simulink model "DIL_26_5_1_2023b"  (R2023b)
settings: Solver=FixedStepAuto  StartTime=0.0  StopTime=inf  FixedStep=0.0005  RelTol=1e-3
PostLoadFcn:
  | modelDir = fileparts(get_param(bdroot,'FileName')); if ~contains([path pathsep],[modelDir pathsep]), addpath(modelDir); end
libraries: Solver_SF x1, slpidlib x1, sl3dlib x1
settings Model: LastModifiedBy=30235
settings SolverCC: AlgebraicLoopSolver=TrustRegion
settings OptimizationCC: DefaultParameterBehavior=Inlined  OptimizeBlockIOStorage=off  EnhancedBackFolding=on  PassReuseOutputArgsThreshold=0  OptimizeDataStoreBuffers=off  BusAssignmentInplaceUpdate=off
settings DebuggingCC: ParameterTunabilityLossMsg=error  UnconnectedInputMsg=warning  UnconnectedOutputMsg=warning  UnconnectedLineMsg=warning  SFUnexpectedBacktrackingDiag=warning  SFNoUnconditionalDefaultTransitionDiag=warning  ArithmeticOperatorsInVariantConditions=warning
settings ModelReferenceCC: EnableRefExpFcnMdlSchedulingChecks=on
settings SFSimCC: MATLABDynamicMemAlloc=off  CustomCodeUndefinedFunction=UseInterfaceOnly
settings RTWCC: GenerateReport=on  BuildConfiguration=Debug  LaunchReport=on  DLArmComputeVersion=19.05
settings CodeAppCC: ForceParamTrailComments=on  OperatorAnnotations=on  MATLABSourceComments=on  EnableCustomComments=on
settings GRTTargetCC: CombineSignalStateStructs=on  SupportVariableSizeSignals=on  MultiInstanceErrorCode=Warning
settings ConfigComp: CovBoundaryAbsTol=1.0e-5

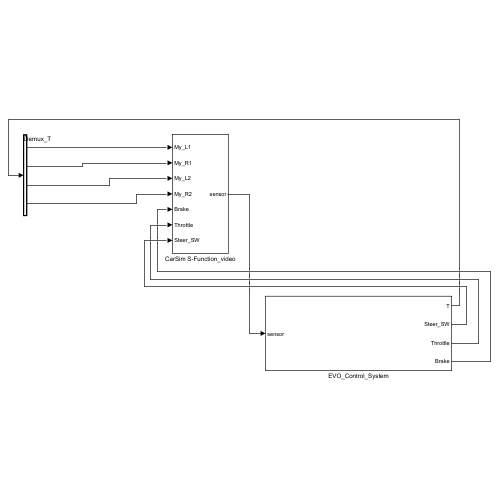
[thumbnail: Simulink's stored preview of the top-level diagram]
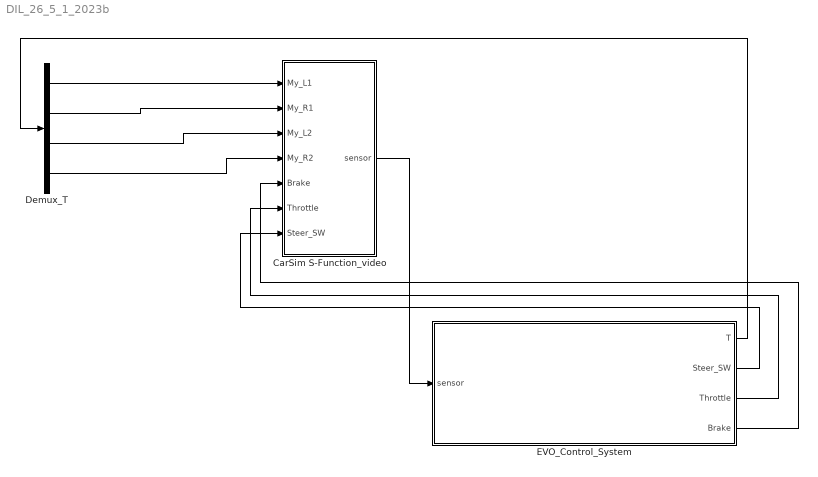
== system DIL_26_5_1_2023b ==
  CarSim S-Function_video : Subsystem
  Demux_T : Demux
  EVO_Control_System : Subsystem
  wires:
  EVO_Control_System/1(T) -> Demux_T/1
  Demux_T/1 -> CarSim S-Function_video/1(My_L1)
  Demux_T/2 -> CarSim S-Function_video/2(My_R1)
  Demux_T/3 -> CarSim S-Function_video/3(My_L2)
  Demux_T/4 -> CarSim S-Function_video/4(My_R2)
  EVO_Control_System/4(Brake) -> CarSim S-Function_video/5(Brake)
  EVO_Control_System/3(Throttle) -> CarSim S-Function_video/6(Throttle)
  EVO_Control_System/2(Steer_SW) -> CarSim S-Function_video/7(Steer_SW)
  CarSim S-Function_video/1(sensor) -> EVO_Control_System/1(sensor)

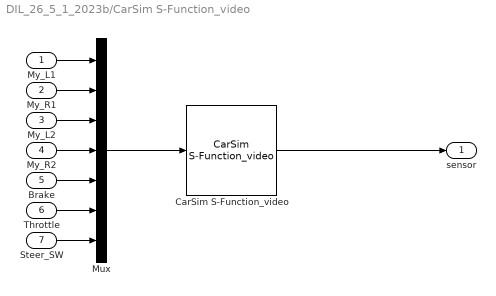
== system DIL_26_5_1_2023b/CarSim S-Function_video ==
  My_L1 : Inport
  My_R1 : Inport  Port=2
  My_L2 : Inport  Port=3
  My_R2 : Inport  Port=4
  Brake : Inport  Port=5
  Throttle : Inport  Port=6
  Steer_SW : Inport  Port=7
  CarSim S-Function_video : Solver_SF/CarSim S-Function_video  Priority=1  SIMFILE=simfile.sim
      settings: SourceProductName=CarSim S-Function
  Mux : Mux  Inputs=7
  sensor : Outport
  wires:
  CarSim S-Function_video/1 -> sensor/1
  My_L1/1 -> Mux/1
  My_R1/1 -> Mux/2
  My_L2/1 -> Mux/3
  My_R2/1 -> Mux/4
  Brake/1 -> Mux/5
  Throttle/1 -> Mux/6
  Steer_SW/1 -> Mux/7
  Mux/1 -> CarSim S-Function_video/1

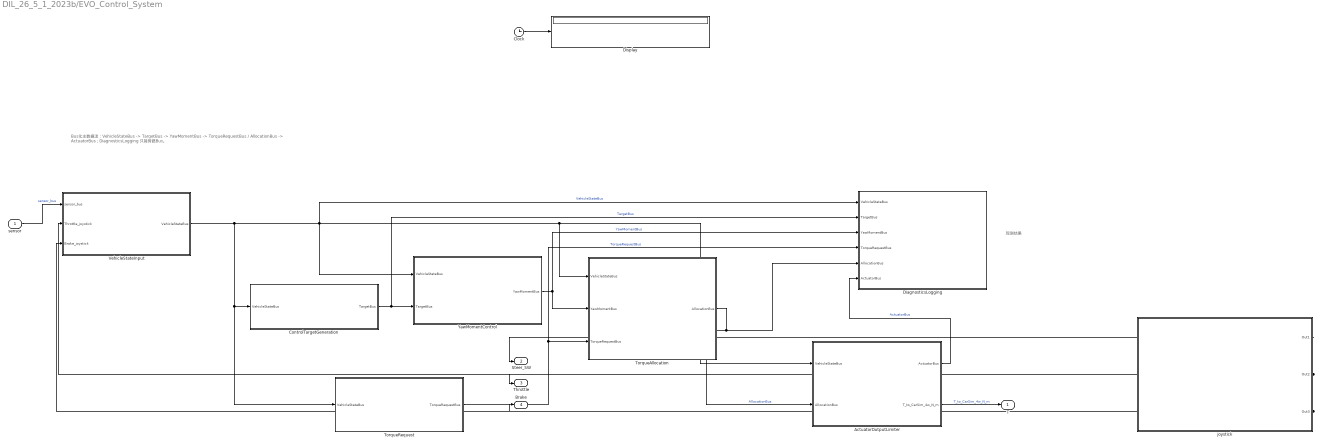
== system DIL_26_5_1_2023b/EVO_Control_System ==
  note: 观测结果
  note: Bus化主数据流：VehicleStateBus -> TargetBus -> YawMomentBus -> TorqueRequestBus / AllocationBus -> ActuatorBus；DiagnosticsLogging 只接旁路Bus。
  sensor : Inport
  ActuatorOutputLimiter : Subsystem  Description=执行器输出限制：统一执行电机转速限扭、最终饱和和传动输出。
  Clock : Clock
  ControlTargetGeneration : Subsystem  Description=控制目标生成：根据车辆状态和转角生成理想侧偏角与理想横摆角速度。
  DiagnosticsLogging : Subsystem  Description=诊断记录：集中显示基础扭矩、DYC 增量、QP 诊断和最终限扭差值。
  Display : Display
  TorqueAllocation : Subsystem  Description=转矩分配：保留简化载荷转移分配和 QP 分配，并通过 TorqueAllocationMode 选择。
  TorqueRequest : Subsystem  Description=基础扭矩请求：根据油门和制动状态生成控制分配层使用的基础扭矩。
  VehicleStateInput : Subsystem  Description=车辆状态输入整理：CarSim sensor 拆分、单位转换、轮胎力估算和基础状态 tag 输出。
  YawMomentControl : Subsystem  Description=横摆力矩控制：保留 PID 与 MPC 两条路径，并通过 YawMomentControlMode 选择。
  joystick : Subsystem
  T : Outport
  Steer_SW : Outport  Port=2
  Throttle : Outport  Port=3
  Brake : Outport  Port=4
  wires:
  sensor/1 -> VehicleStateInput/1(sensor_bus)  "sensor_bus"
  TorqueAllocation/1(AllocationBus) -> ActuatorOutputLimiter/2(AllocationBus), DiagnosticsLogging/5(AllocationBus)  "AllocationBus"
  VehicleStateInput/1(VehicleStateBus) -> ActuatorOutputLimiter/1(VehicleStateBus), TorqueAllocation/1(VehicleStateBus), DiagnosticsLogging/1(VehicleStateBus), YawMomentControl/1(VehicleStateBus), ControlTargetGeneration/1(VehicleStateBus), TorqueRequest/1(VehicleStateBus)  "VehicleStateBus"
  ControlTargetGeneration/1(TargetBus) -> YawMomentControl/2(TargetBus), DiagnosticsLogging/2(TargetBus)  "TargetBus"
  ActuatorOutputLimiter/2(T_to_CarSim_4w_N_m) -> T/1  "T_to_CarSim_4w_N_m"
  ActuatorOutputLimiter/1(ActuatorBus) -> DiagnosticsLogging/6(ActuatorBus)  "ActuatorBus"
  YawMomentControl/1(YawMomentBus) -> DiagnosticsLogging/3(YawMomentBus), TorqueAllocation/2(YawMomentBus)  "YawMomentBus"
  TorqueRequest/1(TorqueRequestBus) -> DiagnosticsLogging/4(TorqueRequestBus), TorqueAllocation/3(TorqueRequestBus)  "TorqueRequestBus"
  Clock/1 -> Display/1
  joystick/1(Out1) -> Steer_SW/1
  joystick/2(Out2) -> Throttle/1, VehicleStateInput/2(Throttle_joystick)
  joystick/3(Out3) -> Brake/1, VehicleStateInput/3(Brake_joystick)

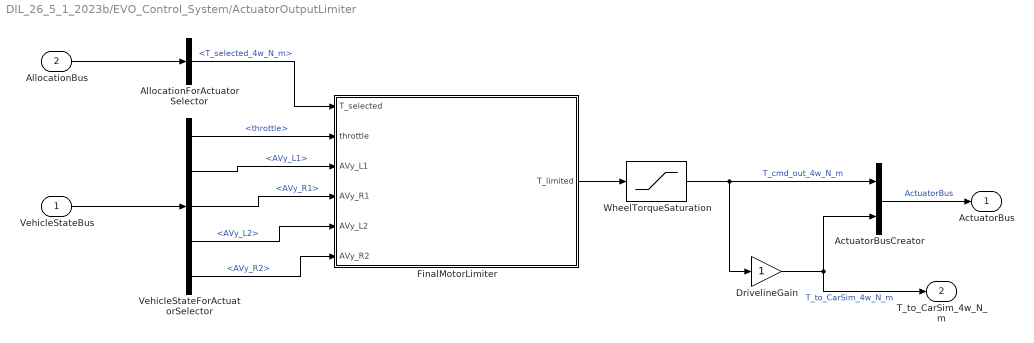
== system DIL_26_5_1_2023b/EVO_Control_System/ActuatorOutputLimiter ==
  VehicleStateBus : Inport
  AllocationBus : Inport  Port=2
  ActuatorBusCreator : BusCreator  Inputs=2
      settings: DisplayOption=signals
  AllocationForActuatorSelector : BusSelector  OutputSignals=T_selected_4w_N_m
  DrivelineGain : Gain
  FinalMotorLimiter : MATLAB Function  TreatAsAtomicUnit=on
  VehicleStateForActuatorSelector : BusSelector  OutputSignals=throttle,AVy_L1,AVy_R1,AVy_L2,AVy_R2
  WheelTorqueSaturation : Saturate  UpperLimit=400  LowerLimit=-400
  ActuatorBus : Outport
  T_to_CarSim_4w_N_m : Outport  Port=2
  wires:
  AllocationBus/1 -> AllocationForActuatorSelector/1
  VehicleStateBus/1 -> VehicleStateForActuatorSelector/1
  AllocationForActuatorSelector/1 -> FinalMotorLimiter/1(T_selected)  "<T_selected_4w_N_m>"
  VehicleStateForActuatorSelector/4 -> FinalMotorLimiter/5(AVy_L2)  "<AVy_L2>"
  VehicleStateForActuatorSelector/2 -> FinalMotorLimiter/3(AVy_L1)  "<AVy_L1>"
  VehicleStateForActuatorSelector/1 -> FinalMotorLimiter/2(throttle)  "<throttle>"
  VehicleStateForActuatorSelector/3 -> FinalMotorLimiter/4(AVy_R1)  "<AVy_R1>"
  VehicleStateForActuatorSelector/5 -> FinalMotorLimiter/6(AVy_R2)  "<AVy_R2>"
  FinalMotorLimiter/1(T_limited) -> WheelTorqueSaturation/1
  WheelTorqueSaturation/1 -> ActuatorBusCreator/1, DrivelineGain/1  "T_cmd_out_4w_N_m"
  DrivelineGain/1 -> ActuatorBusCreator/2, T_to_CarSim_4w_N_m/1  "T_to_CarSim_4w_N_m"
  ActuatorBusCreator/1 -> ActuatorBus/1  "ActuatorBus"

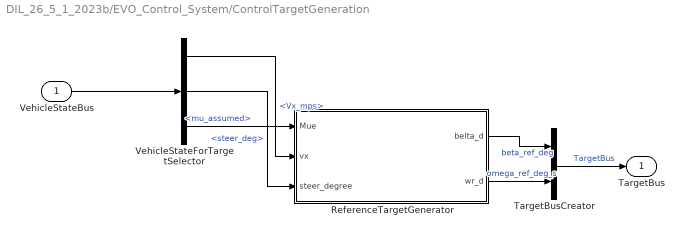
== system DIL_26_5_1_2023b/EVO_Control_System/ControlTargetGeneration ==
  VehicleStateBus : Inport
  ReferenceTargetGenerator : MATLAB Function  TreatAsAtomicUnit=on
  TargetBusCreator : BusCreator  Inputs=2
      settings: DisplayOption=signals
  VehicleStateForTargetSelector : BusSelector  OutputSignals=Vx_mps,steer_deg,mu_assumed
  TargetBus : Outport
  wires:
  VehicleStateForTargetSelector/3 -> ReferenceTargetGenerator/1(Mue)  "<mu_assumed>"
  VehicleStateForTargetSelector/2 -> ReferenceTargetGenerator/3(steer_degree)  "<steer_deg>"
  VehicleStateBus/1 -> VehicleStateForTargetSelector/1
  TargetBusCreator/1 -> TargetBus/1  "TargetBus"
  VehicleStateForTargetSelector/1 -> ReferenceTargetGenerator/2(vx)  "<Vx_mps>"
  ReferenceTargetGenerator/1(belta_d) -> TargetBusCreator/1  "beta_ref_deg"
  ReferenceTargetGenerator/2(wr_d) -> TargetBusCreator/2  "omega_ref_deg_s"

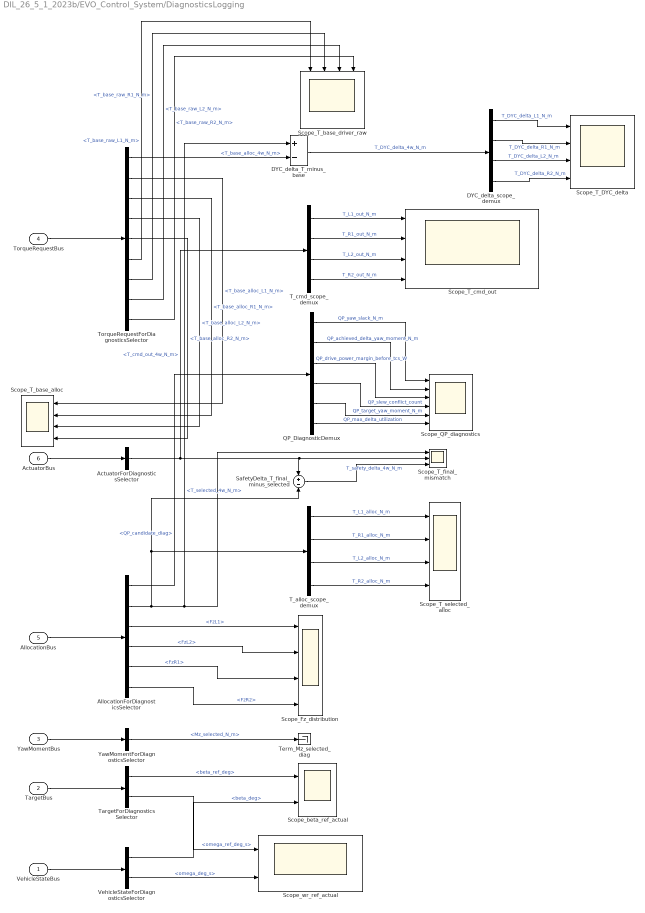
== system DIL_26_5_1_2023b/EVO_Control_System/DiagnosticsLogging ==
  VehicleStateBus : Inport
  TargetBus : Inport  Port=2
  YawMomentBus : Inport  Port=3
  TorqueRequestBus : Inport  Port=4
  AllocationBus : Inport  Port=5
  ActuatorBus : Inport  Port=6
  ActuatorForDiagnosticsSelector : BusSelector  OutputSignals=T_cmd_out_4w_N_m
  AllocationForDiagnosticsSelector : BusSelector  OutputSignals=QP_candidate_diag,T_selected_4w_N_m,FzL1,FzL2,FzR1,FzR2
  DYC_delta_T_minus_base : Sum  Inputs=+-
  DYC_delta_scope_demux : Demux
  QP_DiagnosticDemux : Demux  Outputs=6
  SafetyDelta_T_final_minus_selected : Sum  Inputs=+-
  Scope_Fz_distribution : Scope  NumInputPorts=4
  Scope_QP_diagnostics : Scope  NumInputPorts=6
  Scope_T_DYC_delta : Scope  NumInputPorts=4
  Scope_T_base_alloc : Scope  NumInputPorts=4
  Scope_T_base_driver_raw : Scope  NumInputPorts=4
  Scope_T_cmd_out : Scope  NumInputPorts=4
  Scope_T_final_mismatch : Scope  NumInputPorts=3
  Scope_T_selected_alloc : Scope  NumInputPorts=4
  Scope_beta_ref_actual : Scope  NumInputPorts=2
  Scope_wr_ref_actual : Scope  NumInputPorts=2
  T_alloc_scope_demux : Demux
  T_cmd_scope_demux : Demux
  TargetForDiagnosticsSelector : BusSelector  OutputSignals=beta_ref_deg,omega_ref_deg_s
  Term_Mz_selected_diag : Terminator
  TorqueRequestForDiagnosticsSelector : BusSelector  OutputSignals=T_base_alloc_4w_N_m,T_base_alloc_L1_N_m,T_base_alloc_R1_N_m,T_base_alloc_L2_N_m,T_base_alloc_R2_N_m,T_base_raw_L1_N_m,T_base_raw_R1_N_m,T_base_raw_L2_N_m,T_base_raw_R2_N_m
  VehicleStateForDiagnosticsSelector : BusSelector  OutputSignals=beta_deg,omega_deg_s
  YawMomentForDiagnosticsSelector : BusSelector  OutputSignals=Mz_selected_N_m
  wires:
  QP_DiagnosticDemux/3 -> Scope_QP_diagnostics/3  "QP_drive_power_margin_before_tcs_W"
  ActuatorBus/1 -> ActuatorForDiagnosticsSelector/1
  TorqueRequestBus/1 -> TorqueRequestForDiagnosticsSelector/1
  AllocationForDiagnosticsSelector/3 -> Scope_Fz_distribution/1  "<FzL1>"
  AllocationBus/1 -> AllocationForDiagnosticsSelector/1
  YawMomentBus/1 -> YawMomentForDiagnosticsSelector/1
  T_alloc_scope_demux/1 -> Scope_T_selected_alloc/1  "T_L1_alloc_N_m"
  T_cmd_scope_demux/3 -> Scope_T_cmd_out/3  "T_L2_out_N_m"
  TargetBus/1 -> TargetForDiagnosticsSelector/1
  DYC_delta_scope_demux/1 -> Scope_T_DYC_delta/1  "T_DYC_delta_L1_N_m"
  VehicleStateBus/1 -> VehicleStateForDiagnosticsSelector/1
  TorqueRequestForDiagnosticsSelector/2 -> Scope_T_base_alloc/1  "<T_base_alloc_L1_N_m>"
  DYC_delta_scope_demux/4 -> Scope_T_DYC_delta/4  "T_DYC_delta_R2_N_m"
  TorqueRequestForDiagnosticsSelector/9 -> Scope_T_base_driver_raw/4  "<T_base_raw_R2_N_m>"
  TorqueRequestForDiagnosticsSelector/1 -> DYC_delta_T_minus_base/2  "<T_base_alloc_4w_N_m>"
  TorqueRequestForDiagnosticsSelector/3 -> Scope_T_base_alloc/2  "<T_base_alloc_R1_N_m>"
  VehicleStateForDiagnosticsSelector/1 -> Scope_beta_ref_actual/2  "<beta_deg>"
  TorqueRequestForDiagnosticsSelector/4 -> Scope_T_base_alloc/3  "<T_base_alloc_L2_N_m>"
  VehicleStateForDiagnosticsSelector/2 -> Scope_wr_ref_actual/2  "<omega_deg_s>"
  TorqueRequestForDiagnosticsSelector/5 -> Scope_T_base_alloc/4  "<T_base_alloc_R2_N_m>"
  TorqueRequestForDiagnosticsSelector/6 -> Scope_T_base_driver_raw/1  "<T_base_raw_L1_N_m>"
  TorqueRequestForDiagnosticsSelector/7 -> Scope_T_base_driver_raw/2  "<T_base_raw_R1_N_m>"
  YawMomentForDiagnosticsSelector/1 -> Term_Mz_selected_diag/1  "<Mz_selected_N_m>"
  TorqueRequestForDiagnosticsSelector/8 -> Scope_T_base_driver_raw/3  "<T_base_raw_L2_N_m>"
  ActuatorForDiagnosticsSelector/1 -> SafetyDelta_T_final_minus_selected/1, Scope_T_final_mismatch/2, T_cmd_scope_demux/1  "<T_cmd_out_4w_N_m>"
  AllocationForDiagnosticsSelector/1 -> QP_DiagnosticDemux/1  "<QP_candidate_diag>"
  AllocationForDiagnosticsSelector/2 -> Scope_T_final_mismatch/1, DYC_delta_T_minus_base/1, SafetyDelta_T_final_minus_selected/2, T_alloc_scope_demux/1  "<T_selected_4w_N_m>"
  QP_DiagnosticDemux/5 -> Scope_QP_diagnostics/5  "QP_target_yaw_moment_N_m"
  AllocationForDiagnosticsSelector/4 -> Scope_Fz_distribution/2  "<FzL2>"
  AllocationForDiagnosticsSelector/5 -> Scope_Fz_distribution/3  "<FzR1>"
  AllocationForDiagnosticsSelector/6 -> Scope_Fz_distribution/4  "<FzR2>"
  TargetForDiagnosticsSelector/1 -> Scope_beta_ref_actual/1  "<beta_ref_deg>"
  TargetForDiagnosticsSelector/2 -> Scope_wr_ref_actual/1  "<omega_ref_deg_s>"
  DYC_delta_T_minus_base/1 -> DYC_delta_scope_demux/1  "T_DYC_delta_4w_N_m"
  T_cmd_scope_demux/1 -> Scope_T_cmd_out/1  "T_L1_out_N_m"
  T_cmd_scope_demux/2 -> Scope_T_cmd_out/2  "T_R1_out_N_m"
  T_alloc_scope_demux/2 -> Scope_T_selected_alloc/2  "T_R1_alloc_N_m"
  T_cmd_scope_demux/4 -> Scope_T_cmd_out/4  "T_R2_out_N_m"
  QP_DiagnosticDemux/1 -> Scope_QP_diagnostics/1  "QP_yaw_slack_N_m"
  QP_DiagnosticDemux/2 -> Scope_QP_diagnostics/2  "QP_achieved_delta_yaw_moment_N_m"
  QP_DiagnosticDemux/4 -> Scope_QP_diagnostics/4  "QP_slew_conflict_count"
  QP_DiagnosticDemux/6 -> Scope_QP_diagnostics/6  "QP_max_delta_utilization"
  SafetyDelta_T_final_minus_selected/1 -> Scope_T_final_mismatch/3  "T_safety_delta_4w_N_m"
  T_alloc_scope_demux/3 -> Scope_T_selected_alloc/3  "T_L2_alloc_N_m"
  T_alloc_scope_demux/4 -> Scope_T_selected_alloc/4  "T_R2_alloc_N_m"
  DYC_delta_scope_demux/2 -> Scope_T_DYC_delta/2  "T_DYC_delta_R1_N_m"
  DYC_delta_scope_demux/3 -> Scope_T_DYC_delta/3  "T_DYC_delta_L2_N_m"

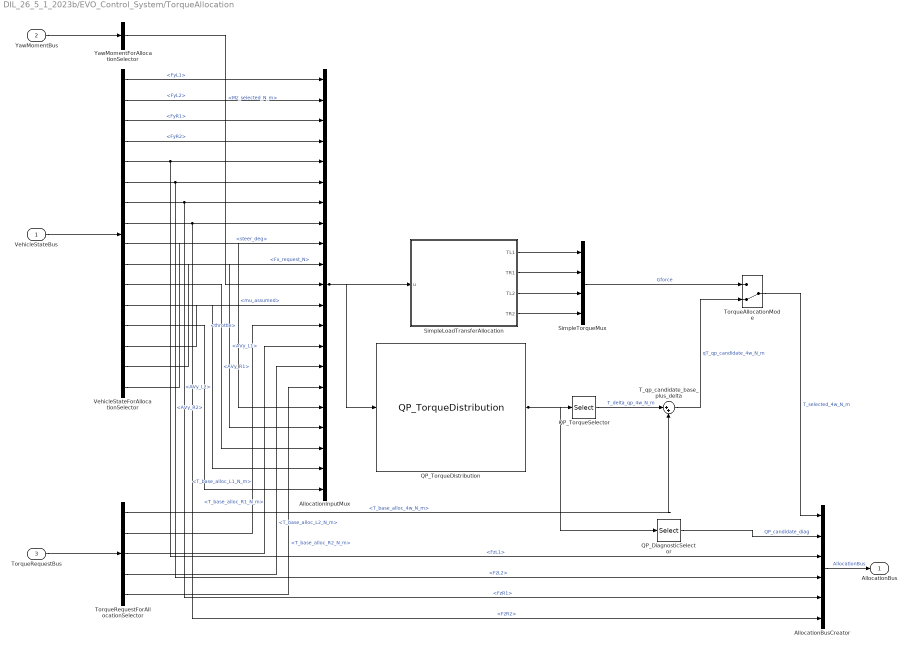
== system DIL_26_5_1_2023b/EVO_Control_System/TorqueAllocation ==
  VehicleStateBus : Inport
  YawMomentBus : Inport  Port=2
  TorqueRequestBus : Inport  Port=3
  AllocationBusCreator : BusCreator  Inputs=6
      settings: DisplayOption=signals
  AllocationInputMux : Mux  Inputs=21
  QP_DiagnosticSelector : Selector  InputPortWidth=10  IndexOptions=Index vector (dialog)  Indices=[5:10]  OutputSizes=6
  QP_TorqueDistribution : M-S-Function  FunctionName=QP_TorqueDistribution
  QP_TorqueSelector : Selector  InputPortWidth=10  IndexOptions=Index vector (dialog)  Indices=[1:4]  OutputSizes=4
  SimpleLoadTransferAllocation : MATLAB Function  TreatAsAtomicUnit=on
  SimpleTorqueMux : Mux
  T_qp_candidate_base_plus_delta : Sum  Inputs=|++
  TorqueAllocationMode : ManualSwitch  CurrentSetting=0
  TorqueRequestForAllocationSelector : BusSelector  OutputSignals=T_base_alloc_4w_N_m,T_base_alloc_L1_N_m,T_base_alloc_R1_N_m,T_base_alloc_L2_N_m,T_base_alloc_R2_N_m
  VehicleStateForAllocationSelector : BusSelector  OutputSignals=FyL1,FyL2,FyR1,FyR2,FzL1,FzL2,FzR1,FzR2,throttle,AVy_L1,AVy_R1,AVy_L2,AVy_R2,mu_assumed,Fx_request_N,steer_deg
  YawMomentForAllocationSelector : BusSelector  OutputSignals=Mz_selected_N_m
  AllocationBus : Outport
  wires:
  TorqueRequestBus/1 -> TorqueRequestForAllocationSelector/1
  VehicleStateBus/1 -> VehicleStateForAllocationSelector/1
  AllocationBusCreator/1 -> AllocationBus/1  "AllocationBus"
  YawMomentBus/1 -> YawMomentForAllocationSelector/1
  VehicleStateForAllocationSelector/11 -> AllocationInputMux/19  "<AVy_R1>"
  YawMomentForAllocationSelector/1 -> AllocationInputMux/11  "<Mz_selected_N_m>"
  TorqueRequestForAllocationSelector/3 -> AllocationInputMux/14  "<T_base_alloc_R1_N_m>"
  VehicleStateForAllocationSelector/4 -> AllocationInputMux/4  "<FyR2>"
  T_qp_candidate_base_plus_delta/1 -> TorqueAllocationMode/2  "qT_qp_candidate_4w_N_m"
  TorqueRequestForAllocationSelector/2 -> AllocationInputMux/13  "<T_base_alloc_L1_N_m>"
  VehicleStateForAllocationSelector/3 -> AllocationInputMux/3  "<FyR1>"
  TorqueRequestForAllocationSelector/1 -> T_qp_candidate_base_plus_delta/2  "<T_base_alloc_4w_N_m>"
  VehicleStateForAllocationSelector/10 -> AllocationInputMux/18  "<AVy_L1>"
  VehicleStateForAllocationSelector/2 -> AllocationInputMux/2  "<FyL2>"
  VehicleStateForAllocationSelector/9 -> AllocationInputMux/17  "<throttle>"
  VehicleStateForAllocationSelector/1 -> AllocationInputMux/1  "<FyL1>"
  TorqueRequestForAllocationSelector/4 -> AllocationInputMux/15  "<T_base_alloc_L2_N_m>"
  VehicleStateForAllocationSelector/5 -> AllocationBusCreator/3, AllocationInputMux/5  "<FzL1>"
  TorqueRequestForAllocationSelector/5 -> AllocationInputMux/16  "<T_base_alloc_R2_N_m>"
  VehicleStateForAllocationSelector/6 -> AllocationBusCreator/4, AllocationInputMux/6  "<FzL2>"
  TorqueAllocationMode/1 -> AllocationBusCreator/1  "T_selected_4w_N_m"
  SimpleTorqueMux/1 -> TorqueAllocationMode/1  "Gforce"
  VehicleStateForAllocationSelector/7 -> AllocationBusCreator/5, AllocationInputMux/7  "<FzR1>"
  VehicleStateForAllocationSelector/8 -> AllocationBusCreator/6, AllocationInputMux/8  "<FzR2>"
  VehicleStateForAllocationSelector/12 -> AllocationInputMux/20  "<AVy_L2>"
  VehicleStateForAllocationSelector/13 -> AllocationInputMux/21  "<AVy_R2>"
  VehicleStateForAllocationSelector/14 -> AllocationInputMux/12  "<mu_assumed>"
  VehicleStateForAllocationSelector/15 -> AllocationInputMux/10  "<Fx_request_N>"
  VehicleStateForAllocationSelector/16 -> AllocationInputMux/9  "<steer_deg>"
  AllocationInputMux/1 -> SimpleLoadTransferAllocation/1(u), QP_TorqueDistribution/1
  SimpleLoadTransferAllocation/1(TL1) -> SimpleTorqueMux/1
  SimpleLoadTransferAllocation/2(TR1) -> SimpleTorqueMux/2
  SimpleLoadTransferAllocation/3(TL2) -> SimpleTorqueMux/3
  SimpleLoadTransferAllocation/4(TR2) -> SimpleTorqueMux/4
  QP_TorqueSelector/1 -> T_qp_candidate_base_plus_delta/1  "T_delta_qp_4w_N_m"
  QP_DiagnosticSelector/1 -> AllocationBusCreator/2  "QP_candidate_diag"
  QP_TorqueDistribution/1 -> QP_TorqueSelector/1, QP_DiagnosticSelector/1

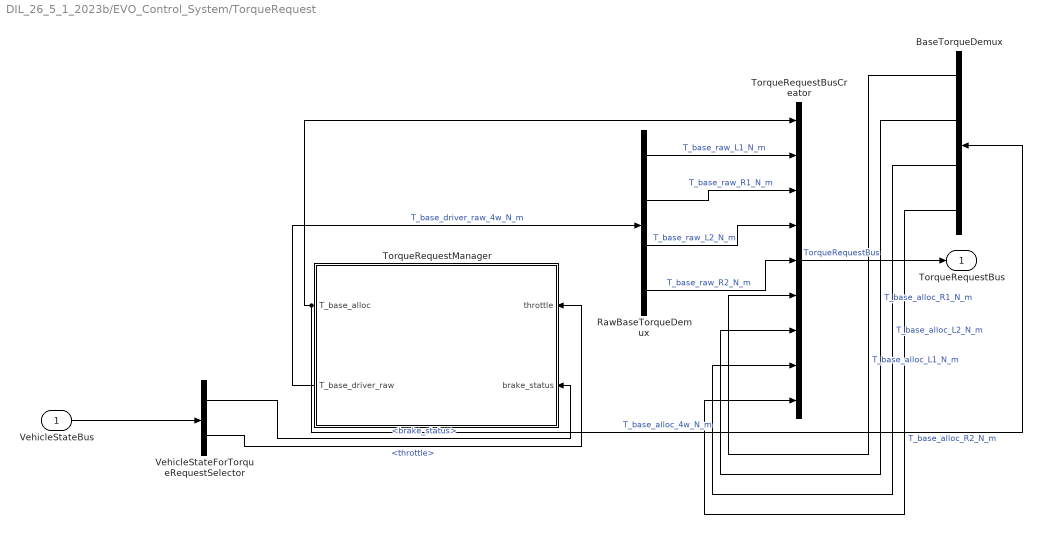
== system DIL_26_5_1_2023b/EVO_Control_System/TorqueRequest ==
  VehicleStateBus : Inport
  BaseTorqueDemux : Demux
  RawBaseTorqueDemux : Demux
  TorqueRequestBusCreator : BusCreator  Inputs=9
      settings: DisplayOption=signals
  TorqueRequestManager : MATLAB Function  TreatAsAtomicUnit=on
  VehicleStateForTorqueRequestSelector : BusSelector  OutputSignals=brake_status,throttle
  TorqueRequestBus : Outport
  wires:
  BaseTorqueDemux/1 -> TorqueRequestBusCreator/6  "T_base_alloc_L1_N_m"
  TorqueRequestManager/1(T_base_alloc) -> BaseTorqueDemux/1, TorqueRequestBusCreator/1  "T_base_alloc_4w_N_m"
  RawBaseTorqueDemux/3 -> TorqueRequestBusCreator/4  "T_base_raw_L2_N_m"
  TorqueRequestBusCreator/1 -> TorqueRequestBus/1  "TorqueRequestBus"
  RawBaseTorqueDemux/2 -> TorqueRequestBusCreator/3  "T_base_raw_R1_N_m"
  RawBaseTorqueDemux/1 -> TorqueRequestBusCreator/2  "T_base_raw_L1_N_m"
  BaseTorqueDemux/2 -> TorqueRequestBusCreator/7  "T_base_alloc_R1_N_m"
  RawBaseTorqueDemux/4 -> TorqueRequestBusCreator/5  "T_base_raw_R2_N_m"
  TorqueRequestManager/2(T_base_driver_raw) -> RawBaseTorqueDemux/1  "T_base_driver_raw_4w_N_m"
  VehicleStateBus/1 -> VehicleStateForTorqueRequestSelector/1
  VehicleStateForTorqueRequestSelector/2 -> TorqueRequestManager/1(throttle)  "<throttle>"
  VehicleStateForTorqueRequestSelector/1 -> TorqueRequestManager/2(brake_status)  "<brake_status>"
  BaseTorqueDemux/4 -> TorqueRequestBusCreator/9  "T_base_alloc_R2_N_m"
  BaseTorqueDemux/3 -> TorqueRequestBusCreator/8  "T_base_alloc_L2_N_m"

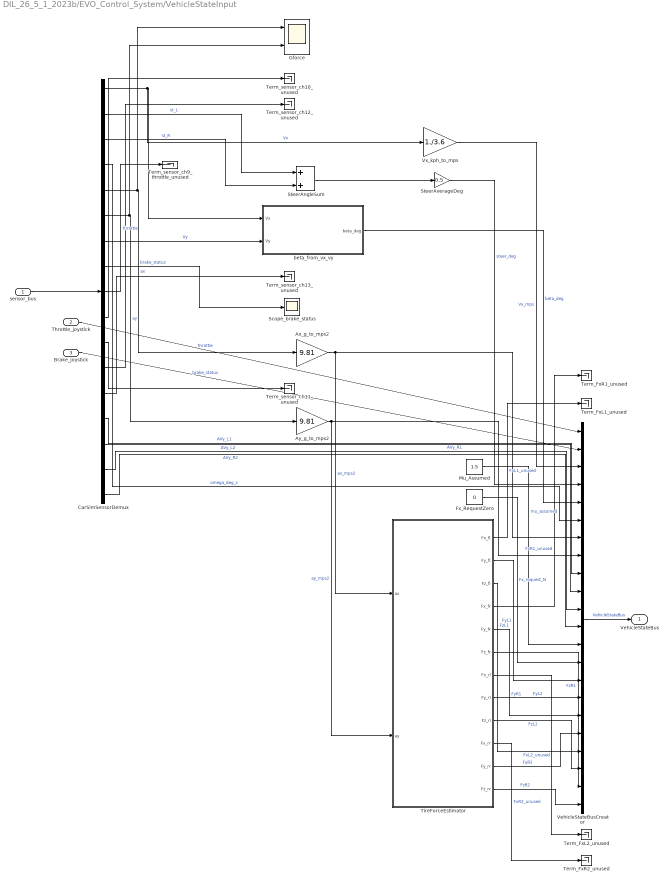
== system DIL_26_5_1_2023b/EVO_Control_System/VehicleStateInput ==
  sensor_bus : Inport
  Throttle_joystick : Inport  Port=2
  Brake_joystick : Inport  Port=3
  Ax_g_to_mps2 : Gain  Gain=9.81
  Ay_g_to_mps2 : Gain  Gain=9.81
  CarSimSensorDemux : Demux  Outputs=17
  Fx_RequestZero : Constant  Value=0
  Gforce : Scope  NumInputPorts=2
  Mu_Assumed : Constant  Value=1.5
  Scope_brake_status : Scope
  SteerAngleSum : Sum
  SteerAverageDeg : Gain  Gain=0.5
  Term_FxL1_unused : Terminator
  Term_FxL2_unused : Terminator
  Term_FxR1_unused : Terminator
  Term_FxR2_unused : Terminator
  Term_sensor_ch10_unused : Terminator
  Term_sensor_ch11_unused : Terminator
  Term_sensor_ch12_unused : Terminator
  Term_sensor_ch13_unused : Terminator
  Term_sensor_ch9_throttle_unused : Terminator
  TireForceEstimator : MATLAB Function  TreatAsAtomicUnit=on
  VehicleStateBusCreator : BusCreator  Inputs=22
      settings: DisplayOption=signals
  Vx_kph_to_mps : Gain  Gain=1./3.6
  beta_from_vx_vy : MATLAB Function  TreatAsAtomicUnit=on
  VehicleStateBus : Outport
  wires:
  CarSimSensorDemux/7 -> beta_from_vx_vy/2(Vy)  "Vy"
  Ay_g_to_mps2/1 -> TireForceEstimator/2(ay), VehicleStateBusCreator/8  "ay_mps2"
  CarSimSensorDemux/6 -> Ay_g_to_mps2/1, Gforce/2  "ay"
  CarSimSensorDemux/5 -> Gforce/1, Ax_g_to_mps2/1  "ax"
  CarSimSensorDemux/4 -> VehicleStateBusCreator/6  "omega_deg_s"
  Ax_g_to_mps2/1 -> VehicleStateBusCreator/7, TireForceEstimator/1(ax)  "ax_mps2"
  CarSimSensorDemux/3 -> SteerAngleSum/2  "st_R"
  CarSimSensorDemux/2 -> SteerAngleSum/1  "st_L"
  CarSimSensorDemux/1 -> Vx_kph_to_mps/1, beta_from_vx_vy/1(Vx)  "Vx"
  sensor_bus/1 -> CarSimSensorDemux/1
  Mu_Assumed/1 -> VehicleStateBusCreator/13  "mu_assumed"
  CarSimSensorDemux/16 -> VehicleStateBusCreator/11  "AVy_L2"
  CarSimSensorDemux/8 -> Scope_brake_status/1  "brake_status"
  SteerAverageDeg/1 -> VehicleStateBusCreator/4  "steer_deg"
  CarSimSensorDemux/17 -> VehicleStateBusCreator/12  "AVy_R2"
  CarSimSensorDemux/10 -> Term_sensor_ch10_unused/1
  Fx_RequestZero/1 -> VehicleStateBusCreator/14  "Fx_request_N"
  CarSimSensorDemux/11 -> Term_sensor_ch11_unused/1
  CarSimSensorDemux/12 -> Term_sensor_ch12_unused/1
  CarSimSensorDemux/13 -> Term_sensor_ch13_unused/1
  SteerAngleSum/1 -> SteerAverageDeg/1
  CarSimSensorDemux/14 -> VehicleStateBusCreator/9  "AVy_L1"
  CarSimSensorDemux/15 -> VehicleStateBusCreator/10  "AVy_R1"
  TireForceEstimator/11(Fy_rr) -> VehicleStateBusCreator/18  "FyR2"
  TireForceEstimator/3(Fz_fl) -> VehicleStateBusCreator/19  "FzL1"
  beta_from_vx_vy/1(beta_deg) -> VehicleStateBusCreator/5  "beta_deg"
  TireForceEstimator/6(Fz_fr) -> VehicleStateBusCreator/21  "FzR1"
  Vx_kph_to_mps/1 -> VehicleStateBusCreator/3  "Vx_mps"
  TireForceEstimator/9(Fz_rl) -> VehicleStateBusCreator/20  "FzL2"
  TireForceEstimator/1(Fx_fl) -> Term_FxL1_unused/1  "FxL1_unused"
  TireForceEstimator/10(Fx_rr) -> Term_FxR2_unused/1  "FxR2_unused"
  TireForceEstimator/2(Fy_fl) -> VehicleStateBusCreator/15  "FyL1"
  TireForceEstimator/12(Fz_rr) -> VehicleStateBusCreator/22  "FzR2"
  TireForceEstimator/4(Fx_fr) -> Term_FxR1_unused/1  "FxR1_unused"
  TireForceEstimator/5(Fy_fr) -> VehicleStateBusCreator/17  "FyR1"
  TireForceEstimator/7(Fx_rl) -> Term_FxL2_unused/1  "FxL2_unused"
  TireForceEstimator/8(Fy_rl) -> VehicleStateBusCreator/16  "FyL2"
  VehicleStateBusCreator/1 -> VehicleStateBus/1  "VehicleStateBus"
  Throttle_joystick/1 -> VehicleStateBusCreator/1  "throttle"
  Brake_joystick/1 -> VehicleStateBusCreator/2  "brake_status"
  CarSimSensorDemux/9 -> Term_sensor_ch9_throttle_unused/1  "throttle"

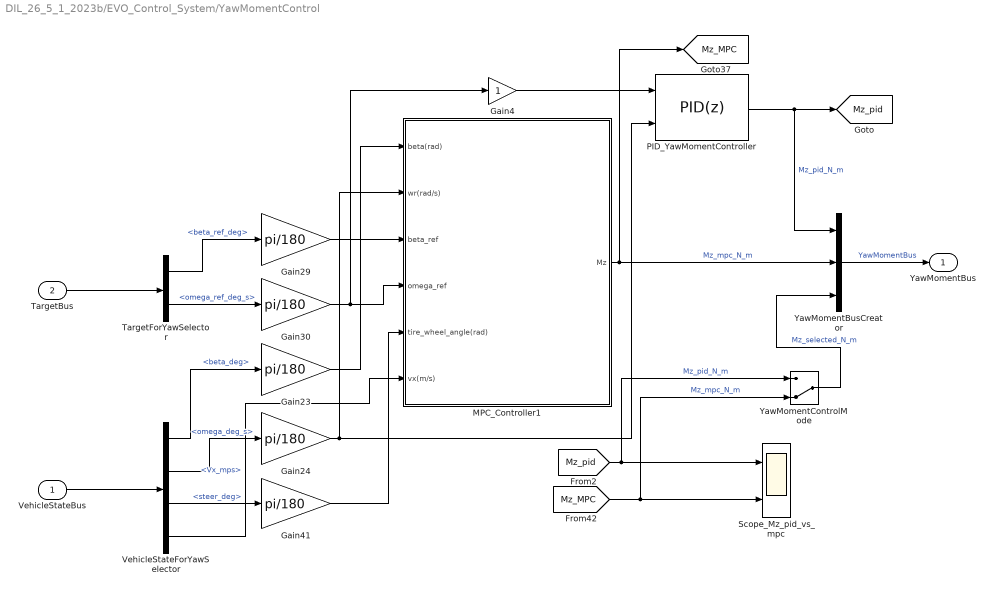
== system DIL_26_5_1_2023b/EVO_Control_System/YawMomentControl ==
  VehicleStateBus : Inport
  TargetBus : Inport  Port=2
  Gain{23..24,29..30,41} (5 alike) : Gain  Gain=pi/180
  Gain4 : Gain
  MPC_Controller1 : Subsystem
  PID_YawMomentController : slpidlib/PID Controller (2DOF)  Controller=PID  Form=Parallel  TimeDomain=Discrete-time  UseExternalTs=off  SampleTime=-1  IntegratorMethod=Forward Euler  FilterMethod=Forward Euler  ControllerParametersSource=internal  P=6000  I=200  UseKiTs=off  D=0  N=100  UseFilter=on  b=1  c=1  TunerSelectOption=Transfer Function Based (PID Tuner App)  InitialConditionSource=internal  InitialConditionForIntegrator=0  InitialConditionForFilter=0  DifferentiatorICPrevScaledInput=0  ExternalReset=none  TrackingMode=off  Kt=1  LimitOutput=off  SatLimitsSource=internal  UpperSaturationLimit=inf  LowerSaturationLimit=-inf  LinearizeAsGain=on  AntiWindupMode=none  Kb=1  LimitIntegrator=off  UpperIntegratorSaturationLimit=inf  LowerIntegratorSaturationLimit=-inf  POutMin=[]  POutMax=[]  IOutMin=[]  IOutMax=[]  DOutMin=[]  DOutMax=[]  NOutMin=[]  NOutMax=[]  bOutMin=[]  bOutMax=[]  cOutMin=[]  cOutMax=[]  SumOutMin=[]  SumOutMax=[]  SaturationOutMin=[]  SaturationOutMax=[]  PParamMin=[]  PParamMax=[]  IParamMin=[]  IParamMax=[]  DParamMin=[]  DParamMax=[]  NParamMin=[]  NParamMax=[]  bParamMin=[]  bParamMax=[]  cParamMin=[]  cParamMax=[]  KbParamMin=[]  KbParamMax=[]  KtParamMin=[]  KtParamMax=[]  KbOutMin=[]  KbOutMax=[]  KtOutMin=[]  KtOutMax=[]  IntegratorOutMin=[]  IntegratorOutMax=[]  FilterOutMin=[]  FilterOutMax=[]  SumI1OutMin=[]  SumI1OutMax=[]  SumI2OutMin=[]  SumI2OutMax=[]  SumI3OutMin=[]  SumI3OutMax=[]  SumI4OutMin=[]  SumI4OutMax=[]  SumDOutMin=[]  SumDOutMax=[]  Sum1OutMin=[]  Sum1OutMax=[]  Sum2OutMin=[]  Sum2OutMax=[]  Sum3OutMin=[]  Sum3OutMax=[]  DifferentiatorOutMin=[]  DifferentiatorOutMax=[]  FilterDiffOutCoefMin=[]  FilterDiffOutCoefMax=[]  ReciprocalOutMin=[]  ReciprocalOutMax=[]  SumDenOutMin=[]  SumDenOutMax=[]  SumNumOutMin=[]  SumNumOutMax=[]  DivideOutMin=[]  DivideOutMax=[]  UdiffTsProdOutMin=[]  UdiffTsProdOutMax=[]  NTsProdOutMin=[]  NTsProdOutMax=[]  UintegralTsProdOutMin=[]  UintegralTsProdOutMax=[]  UngainTsProdOutMin=[]  UngainTsProdOutMax=[]  ClampingZeroOutDataTypeStr=Inherit: Inherit via back propagation  ClampingZeroOutMin=[]  ClampingZeroOutMax=[]  FilterDenConstantOutDataTypeStr=Inherit: Inherit via back propagation  FilterDenConstantOutMin=[]  FilterDenConstantOutMax=[]  PCopyOutDataTypeStr=Inherit: Inherit via back propagation  PCopyOutMin=[]  PCopyOutMax=[]  NCopyOutDataTypeStr=Inherit: Inherit via back propagation  NCopyOutMin=[]  NCopyOutMax=[]  IntegratorContinuousStateAttributes=''  IntegratorStateMustResolveToSignalObject=off  IntegratorRTWStateStorageClass=Auto  FilterContinuousStateAttributes=''  FilterStateMustResolveToSignalObject=off  FilterRTWStateStorageClass=Auto  ParallelPVariant=InternalParameters  IdealPVariant=Disabled  IVariant=InternalParameters  DVariant=InternalParameters  bVariant=InternalParameters  cVariant=InternalParameters  IntegratorVariant=Discrete  SatVariant=Disabled  AWVariant=Passthrough  PCopyVariant=Disabled  TRVariant=Disabled  FdbkBlocksVariant=Forward  IdealPFdbkVariant=Disabled  SatFdbkVariant=Disabled  DerivativeFilterVariant=ForwardEulerFilter  NVariant=InternalParameters  NCopyVariant=Disabled  FilterICVariant=InternalICsFilter  IntegratorICVariant=InternalICs  ExternalResetVariant=Disabled  TRSumVariant=Passthrough  SumFdbkVariant=Disabled  SumVariant=Sum_PID  TsampFilterVariant=InternalTs  TsampNgainVariant=Passthrough  TsampIntegralVariant=Disabled_SignalSpec  ExternalSaturationOutDataTypeStr=Inherit: Same as second input
  Scope_Mz_pid_vs_mpc : Scope  NumInputPorts=2
  TargetForYawSelector : BusSelector  OutputSignals=beta_ref_deg,omega_ref_deg_s
  VehicleStateForYawSelector : BusSelector  OutputSignals=beta_deg,omega_deg_s,steer_deg,Vx_mps
  YawMomentBusCreator : BusCreator  Inputs=3
      settings: DisplayOption=signals
  YawMomentControlMode : ManualSwitch  CurrentSetting=0
  YawMomentBus : Outport
  tag scope: Mz_MPC=global, Mz_pid=global
  wires:
  TargetBus/1 -> TargetForYawSelector/1
  VehicleStateBus/1 -> VehicleStateForYawSelector/1
  VehicleStateForYawSelector/1 -> Gain23/1  "<beta_deg>"
  TargetForYawSelector/1 -> Gain29/1  "<beta_ref_deg>"
  VehicleStateForYawSelector/2 -> Gain24/1  "<omega_deg_s>"
  TargetForYawSelector/2 -> Gain30/1  "<omega_ref_deg_s>"
  VehicleStateForYawSelector/3 -> Gain41/1  "<steer_deg>"
  VehicleStateForYawSelector/4 -> MPC_Controller1/6(vx(m/s))  "<Vx_mps>"
  Gain29/1 -> MPC_Controller1/3(beta_ref)
  Gain30/1 -> MPC_Controller1/4(omega_ref), Gain4/1
  Gain23/1 -> MPC_Controller1/1(beta(rad))
  Gain24/1 -> MPC_Controller1/2(wr(rad/s)), PID_YawMomentController/2
  Gain41/1 -> MPC_Controller1/5(tire_wheel_angle(rad))
  Gain4/1 -> PID_YawMomentController/1
  MPC_Controller1/1(Mz) -> YawMomentBusCreator/2, [Mz_MPC]  "Mz_mpc_N_m"
  [Mz_pid] -> YawMomentControlMode/1, Scope_Mz_pid_vs_mpc/1  "Mz_pid_N_m"
  [Mz_MPC] -> Scope_Mz_pid_vs_mpc/2, YawMomentControlMode/2  "Mz_mpc_N_m"
  PID_YawMomentController/1 -> YawMomentBusCreator/1, [Mz_pid]  "Mz_pid_N_m"
  YawMomentControlMode/1 -> YawMomentBusCreator/3  "Mz_selected_N_m"
  YawMomentBusCreator/1 -> YawMomentBus/1  "YawMomentBus"

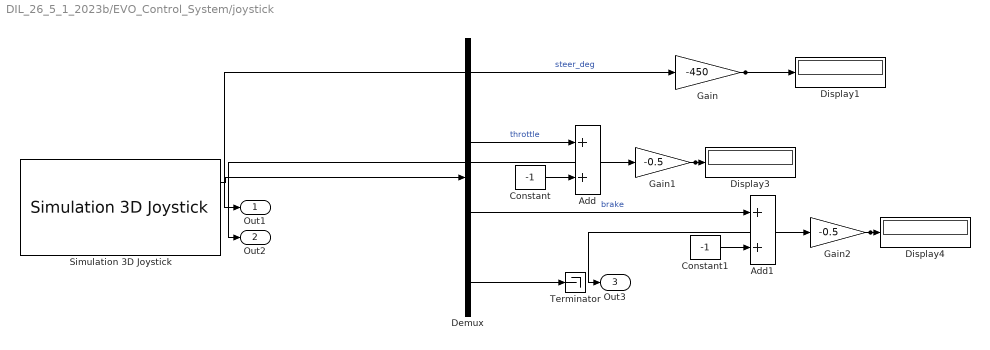
== system DIL_26_5_1_2023b/EVO_Control_System/joystick ==
  Add : Sum
  Add1 : Sum
  Constant : Constant  Value=-1
  Constant1 : Constant  Value=-1
  Demux : Demux
  Display1 : Display
  Display3 : Display
  Display4 : Display
  Gain : Gain  Gain=-450
  Gain1 : Gain  Gain=-0.5
  Gain2 : Gain  Gain=-0.5
  Simulation 3D Joystick : sl3dlib/Simulation 3D/Hardware Interface/Simulation 3D Joystick  joyid=1  adjustports=on  forcefeed=off
  Terminator : Terminator
  Out1 : Outport
  Out2 : Outport  Port=2
  Out3 : Outport  Port=3
  wires:
  Demux/4 -> Terminator/1
  Demux/3 -> Add1/1  "brake"
  Gain2/1 -> Display4/1, Out3/1
  Gain1/1 -> Display3/1, Out2/1
  Constant1/1 -> Add1/2
  Add1/1 -> Gain2/1
  Demux/1 -> Gain/1  "steer_deg"
  Add/1 -> Gain1/1
  Gain/1 -> Display1/1, Out1/1
  Demux/2 -> Add/1  "throttle"
  Simulation 3D Joystick/1 -> Demux/1
  Constant/1 -> Add/2

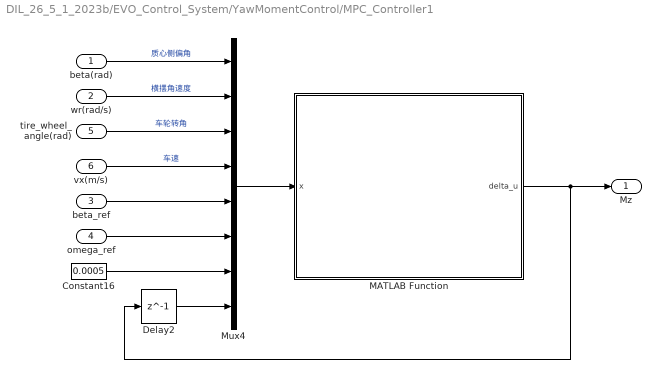
== system DIL_26_5_1_2023b/EVO_Control_System/YawMomentControl/MPC_Controller1 ==
  beta(rad) : Inport
  wr(rad/s) : Inport  Port=2
  beta_ref : Inport  Port=3
  omega_ref : Inport  Port=4
  tire_wheel_angle(rad) : Inport  Port=5
  vx(m/s) : Inport  Port=6
  Constant16 : Constant  Value=0.0005
  Delay2 : Delay  DelayLength=1
  MATLAB Function : MATLAB Function  TreatAsAtomicUnit=on
  Mux4 : Mux  Inputs=8
  Mz : Outport
  wires:
  beta(rad)/1 -> Mux4/1  "质心侧偏角"
  tire_wheel_angle(rad)/1 -> Mux4/3  "车轮转角"
  vx(m/s)/1 -> Mux4/4  "车速"
  Mux4/1 -> MATLAB Function/1(x)
  wr(rad/s)/1 -> Mux4/2  "横摆角速度"
  beta_ref/1 -> Mux4/5
  omega_ref/1 -> Mux4/6
  Delay2/1 -> Mux4/8
  Constant16/1 -> Mux4/7
  MATLAB Function/1(delta_u) -> Delay2/1, Mz/1

== matlab function DIL_26_5_1_2023b/EVO_Control_System/VehicleStateInput/beta_from_vx_vy ==
  data: Vx input; beta_deg output; Vy input
function beta_deg = beta_from_vx_vy(Vx, Vy)
% 根据CarSim导出的纵向/横向速度估算质心侧偏角。
% Vx与Vy只要单位一致即可，atan2比值不会受km/h或m/s影响。
vx_min = 0.1; % 低速时侧偏角噪声很大，直接输出0作为保护。
if ~isfinite(Vx) || ~isfinite(Vy)
    beta_deg = 0;
    return;
end
if abs(Vx) < vx_min
    beta_deg = 0;
else
    beta_deg = atan2(Vy, Vx) * 180/pi;
end
end

== matlab function DIL_26_5_1_2023b/EVO_Control_System/ControlTargetGeneration/ReferenceTargetGenerator ==
  data: Mue input; belta_d output; vx input; wr_d output; steer_degree input
function [belta_d,wr_d] = fcn(Mue,vx,steer_degree)
% 根据二自由度车辆模型计算理想质心侧偏角和横摆角速度。
% 输入单位：vx为m/s，steer_degree为deg，Mue为路面附着系数。

veh = DYC_vehicle_params;
l = veh.L;       % 轴距，m
lf = veh.lf;     % 质心到前轴距离，m
lr = veh.lr;     % 质心到后轴距离，m
m = veh.m;       % 整车质量，kg
mu = Mue;        % 路面附着系数
g = 9.81;        % 重力加速度，m/s^2
kf = veh.Cf;     % 前轴等效侧偏刚度，N/rad
kr = veh.Cr;     % 后轴等效侧偏刚度，N/rad
Kf = (m/l^2)*((lf/kr)-(lr/kf));
vx_min = 0.5;
vx_safe = max(abs(vx), vx_min); % 低速保护，避免理想响应公式除以接近0的车速。

% 未限幅理想值：gama1为横摆角速度rad/s，belta1为侧偏角rad。
gama1 = ((vx_safe*(steer_degree*pi/180))/(l*(1+Kf*vx_safe^2)));
belta1 = ((lr/vx_safe^2 + (m*lf)/(kr*l))*(vx_safe^2/(l*(1+Kf*vx_safe^2)))*(steer_degree*pi/180));
% 附着约束上限：由路面Mu和重力加速度限制理想响应幅值。
gama2 = abs((mu*g)/vx_safe); % rad/s
belta2 = abs(mu*g*((lr/vx_safe^2)+(m*lf)/(kr*l))); % rad

% 保留理想响应符号，同时把幅值限制在附着允许范围内。
if (gama1 > 0)
    C = [gama1*180/pi gama2*180/pi];
    wr_d = min(C);
else
    C = [gama1*180/pi -gama2*180/pi];
    wr_d = max(C);
end
if (belta1 > 0)
    D = [belta1*180/pi belta2*180/pi];
    belta_d = min(D);  % deg
else
    D = [belta1*180/pi -belta2*180/pi];
    belta_d = max(D);  % deg
end
end

== matlab function DIL_26_5_1_2023b/EVO_Control_System/VehicleStateInput/TireForceEstimator ==
  data: ax input; Fx_fl output; ay input; Fy_fl output; Fz_fl output; Fx_fr output; Fy_fr output; Fz_fr output; Fx_rl output; Fy_rl output; Fz_rl output; Fx_rr output; Fy_rr output; Fz_rr output
function [Fx_fl, Fy_fl, Fz_fl, Fx_fr, Fy_fr, Fz_fr, Fx_rl, Fy_rl, Fz_rl, Fx_rr, Fy_rr, Fz_rr] = calculateTireForces(ax, ay)
% 根据质心处纵向/横向加速度估算四轮垂向载荷。
% ax和ay的单位应为m/s^2，上游Gain已将CarSim的g单位转换为m/s^2。
% 该块当前只给DYC/QP提供Fz估计，Fx/Fy输出保持为0。

veh = DYC_vehicle_params;
m = veh.m;      % 整车质量，kg
g = 9.81;       % 重力加速度，m/s^2
Lf = veh.lf;    % 质心到前轴距离，m
Lr = veh.lr;    % 质心到后轴距离，m
L = veh.L;      % 轴距，m
h = 0.3;        % 质心高度，m；当前模型保留原估计值。
tf = veh.tf;    % 前轮距，m
tr = veh.tr;    % 后轮距，m

% 纵向载荷转移：ax为正时，载荷由前轴向后轴转移。
Fzf = m*g*Lr/L - m*ax*h/L;
Fzr = m*g*Lf/L + m*ax*h/L;

% 横向载荷转移：沿用当前模型约定，ay为正时右侧车轮增载、左侧车轮减载。
% 先按动态前/后轴载荷分别计算该轴内部的左右载荷转移量。
dFzf_lat = (Fzf/g) * ay * h / tf;
dFzr_lat = (Fzr/g) * ay * h / tr;

% 四轮垂向载荷。
Fz_fl = Fzf/2 - dFzf_lat;
Fz_fr = Fzf/2 + dFzf_lat;
Fz_rl = Fzr/2 - dFzr_lat;
Fz_rr = Fzr/2 + dFzr_lat;

% 物理保护：垂向载荷不允许为负，并将总载荷归一回整车重量。
Fz = max([Fz_fl; Fz_fr; Fz_rl; Fz_rr], 0);
sumFz = sum(Fz);
targetTotal = m*g;
if sumFz > 1e-6
    Fz = Fz * targetTotal / sumFz;
end

Fz_fl = Fz(1);
Fz_fr = Fz(2);
Fz_rl = Fz(3);
Fz_rr = Fz(4);

% 当前块只估算垂向载荷，纵向/横向轮胎力暂不在这里估算。
Fx_fl = 0;
Fy_fl = 0;
Fx_fr = 0;
Fy_fr = 0;
Fx_rl = 0;
Fy_rl = 0;
Fx_rr = 0;
Fy_rr = 0;
end

== matlab function DIL_26_5_1_2023b/EVO_Control_System/TorqueRequest/TorqueRequestManager ==
  data: throttle input; T_base_alloc output; brake_status input; T_base_driver_raw output
function [T_base_alloc, T_base_driver_raw] = torque_request_manager(throttle, brake_status)
% 根据油门和制动状态生成分配层基础扭矩，同时保留原始踏板需求。
% T_base_alloc用于控制分配，T_base_driver_raw只用于诊断和对比。
[T_base_alloc, T_base_driver_raw] = DYC_torque_request_manager(throttle, brake_status);
end

== matlab function DIL_26_5_1_2023b/EVO_Control_System/ActuatorOutputLimiter/FinalMotorLimiter ==
  data: T_selected input; T_limited output; throttle input; AVy_L1 input; AVy_R1 input; AVy_L2 input; AVy_R2 input
function T_limited = final_motor_limiter(T_selected, throttle, AVy_L1, AVy_R1, AVy_L2, AVy_R2)
% 对最终四轮扭矩统一执行电机转速限扭和总正驱动功率限扭。
% T_selected按[L1; R1; L2; R2]排列，AVy_*为各轮角速度/轮速反馈通道。
wheelRpm = [AVy_L1; AVy_R1; AVy_L2; AVy_R2];
% 具体限扭逻辑放在共享MATLAB函数中，保证模型块和单元测试使用同一实现。
T_limited = DYC_apply_motor_limits(T_selected, throttle, wheelRpm);
end

== matlab function DIL_26_5_1_2023b/EVO_Control_System/TorqueAllocation/SimpleLoadTransferAllocation ==
  data: u input; TL1 output; TR1 output; TL2 output; TR2 output
function [TL1, TR1, TL2, TR2] = Gforce_TorqueDistribution(u)
% 输出踏板基础扭矩叠加DYC附加扭矩，电机限扭由后端统一处理。
% 输入u沿用QP接口顺序，输出轮序为[L1, R1, L2, R2]。
torqueCommand = DYC_simple_load_transfer_distribution(u);
TL1 = torqueCommand(1);
TR1 = torqueCommand(2);
TL2 = torqueCommand(3);
TR2 = torqueCommand(4);
end

== matlab function DIL_26_5_1_2023b/EVO_Control_System/YawMomentControl/MPC_Controller1/MATLAB Function ==
  data: x input size=[8,1]; delta_u output
function delta_u = fcn(x)
% 增量式MPC横摆力矩控制器，输出绝对附加横摆力矩Mz。
% 输入x = [beta; omega; delta; vx; beta_ref; omega_ref; T; Mz_last]。
Np = 8;     % 预测时域
Nc = 5;     % 控制时域
x_num = 2;  % 状态量个数：质心侧偏角和横摆角速度

% 车辆参数。
veh = DYC_vehicle_params;
lf = veh.lf;    % 质心到前轴距离，m
lr = veh.lr;    % 质心到后轴距离，m
m = veh.m;      % 整车质量，kg
Iz = veh.Iz;    % 横摆转动惯量，kg*m^2
Cf = veh.Cf;    % 前轴等效侧偏刚度，N/rad
Cr = veh.Cr;    % 后轴等效侧偏刚度，N/rad

% 输入量。
beta = x(1);
omega = x(2);
delta = x(3);
u = x(4);
u_min = 0.5;
u = max(abs(u), u_min); % 低速保护，避免二自由度模型中除以接近0的车速。
u_k_1 = x(8);
ksi = [beta; omega; u_k_1];

% 二自由度车辆模型。侧偏刚度采用负值符号约定。
a11 = (Cf + Cr)/(m*u);
a12 = (Cf*lf - Cr*lr)/(m*u^2) - 1;
a21 = (Cf*lf - Cr*lr)/Iz;
a22 = (lf^2*Cf + lr^2*Cr)/(Iz*u);
b11 = -Cf/(m*u);
b21 = -lf*Cf/Iz;
A = [a11, a12; a21, a22];
B = [0; 1/Iz];
Bcd = [b11; b21];

T = x(7);
nx = length(A);
G = T*A + eye(nx);
Hd = T*B;
Bd = T*Bcd;

% 增广系统：优化量为附加横摆力矩增量，输出量为绝对附加横摆力矩。
A_ = [G, Hd; zeros(1,2), 1];
B_ = [Hd; 1];
C_ = [eye(2), zeros(2,1)];
Bd_ = [Bd; 0];

% Sc描述当前状态在预测时域内对输出的自由响应。
Sc = zeros(Np*x_num, x_num + 1);
for i = 1:Np
    Sc((x_num*(i-1)+1):x_num*i, :) = C_*(A_^i);
end

% Sd描述前轮转角扰动在预测时域内的累积影响。
tmp = zeros(x_num,1);
Sd = zeros(Np*x_num,1);
for i = 1:Np
    tmp = tmp + C_*(A_^(i-1))*Bd_;
    Sd((x_num*(i-1)+1):x_num*i) = tmp;
end

% Su描述未来控制增量序列对预测输出的影响。
Su = zeros(Np*x_num, Nc);
for i = 1:Np
    Su_tmp = zeros(x_num, Nc);
    for j = 1:Nc
        if j <= i
            Su_tmp(:,j) = C_*(A_^(i-j))*B_;
        end
    end
    Su((x_num*(i-1)+1):x_num*i, :) = Su_tmp;
end

% 当前权重只重点跟踪横摆角速度，侧偏角权重保留为0。
Q = zeros(Np*x_num, Np*x_num);
Qi = [0, 0; 0, 10];
for i = 1:Np
    idx = (x_num*(i-1)+1):x_num*i;
    Q(idx, idx) = Qi;
end

beta_ref = x(5);
omega_ref = x(6);
Ri = [beta_ref; omega_ref];
Ref = zeros(Np*x_num,1);
for i = 1:Np
    Ref((x_num*(i-1)+1):x_num*i) = Ri;
end

% 构造无约束二次型并求解第一拍控制增量。
E = Sc*ksi + Sd*delta - Ref;
R = 0.0003*eye(Nc);
Hqp = 2*(Su'*Q*Su + R);
Hqp = Hqp + 1e-9*eye(Nc);
Gqp = 2*E'*Q*Su;

delta_u_arr = -(Hqp \ Gqp');
delta_mz = delta_u_arr(1);

% 为保持外部端口兼容，输出变量名仍为delta_u；其物理含义为绝对附加横摆力矩Mz。
delta_u = u_k_1 + delta_mz;
delta_u = max(-1000, delta_u);
delta_u = min(1000, delta_u);
end
